simulink model "lab4"  (R2018b)
settings: Solver=ode4  StartTime=0.0  StopTime=10.0  FixedStep=0.01  RelTol=1e-3
values from neighbouring files (symbols this model uses):
  A0 = double(A0)    [scriptlab4.m]    (also in scriptlab5.m = A + B*F0; scriptlab7.m = A + B*F0)
  Ac = double(Ac)    [scriptlab4.m]    (also in scriptlab7.m = J + H*F*M)
  B0 = double(B0)    [scriptlab4.m]
  Bc = double(Bc)    [scriptlab4.m]    (also in scriptlab7.m = K + H*F*N)
  C0 = double(C0)    [scriptlab4.m]
  Cc = double(Cc)    [scriptlab4.m]
settings Model: Creator=grecu  LastModifiedBy=grecu

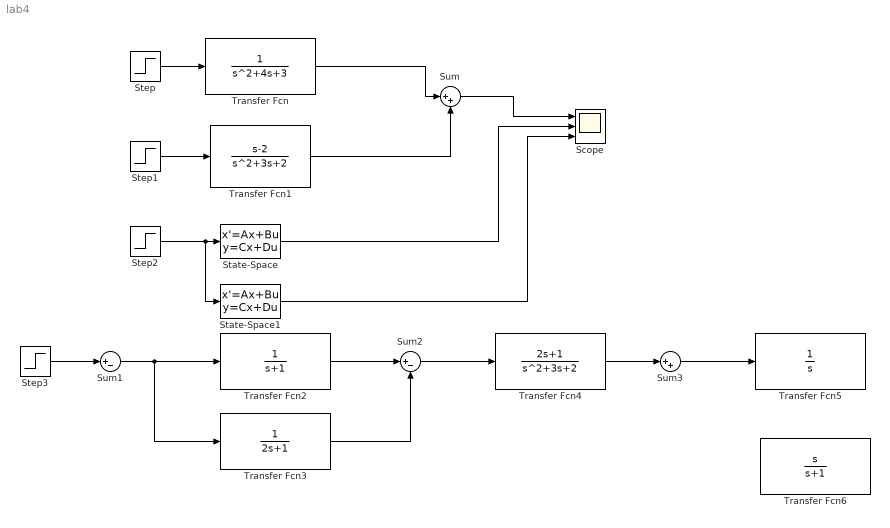
== system lab4 ==
  Scope : Scope  NumInputPorts=3
  State-Space : StateSpace  A=Ac  B=Bc  C=Cc  D=[0, 0]  InitialCondition=0
  State-Space1 : StateSpace  A=A0  B=B0  C=C0  D=[0, 0]  InitialCondition=0
  Step : Step  SampleTime=0
  Step1 : Step  After=-2  SampleTime=0
  Step2 : Step  After=[1;-2]  SampleTime=0
  Step3 : Step  SampleTime=0
  Sum : Sum  Inputs=|++
  Sum1 : Sum  Inputs=|+-
  Sum2 : Sum  Inputs=|+-
  Sum3 : Sum  Inputs=|++
  Transfer Fcn : TransferFcn  Denominator=[1 4 3]
  Transfer Fcn1 : TransferFcn  Numerator=[1 -2]  Denominator=[1 3 2]
  Transfer Fcn2 : TransferFcn  Denominator=[1 1]
  Transfer Fcn3 : TransferFcn  Denominator=[2 1]
  Transfer Fcn4 : TransferFcn  Numerator=[2 1]  Denominator=[1 3 2]
  Transfer Fcn5 : TransferFcn  Denominator=[1 0]
  Transfer Fcn6 : TransferFcn  Numerator=[1 0]  Denominator=[1 1]
  wires:
  Step1/1 -> Transfer Fcn1/1
  Step/1 -> Transfer Fcn/1
  Transfer Fcn/1 -> Sum/1
  Transfer Fcn1/1 -> Sum/2
  Sum/1 -> Scope/1
  Step2/1 -> State-Space1/1, State-Space/1
  State-Space/1 -> Scope/2
  State-Space1/1 -> Scope/3
  Step3/1 -> Sum1/1
  Sum1/1 -> Transfer Fcn3/1, Transfer Fcn2/1
  Transfer Fcn2/1 -> Sum2/1
  Transfer Fcn3/1 -> Sum2/2
  Sum2/1 -> Transfer Fcn4/1
  Transfer Fcn4/1 -> Sum3/1
  Sum3/1 -> Transfer Fcn5/1
